simulink model "SpheroGigETracking"  (R2017b)
settings: Solver=FixedStepAuto  StartTime=0.0  StopTime=inf  RelTol=1e-3
undefined symbols (not defined in the file or in its folder): DeviceSpecific, gray, Rec, SDTV, videoinput
libraries: visionstatistics x2, dspnetwork x2, visionconversions x1, visiontextngfix x1, sphero_lib x1, imaqlib x1
settings Model: Creator=Michael  LastModifiedBy=Admin
settings CodeAppCC: StateflowObjectComments=on

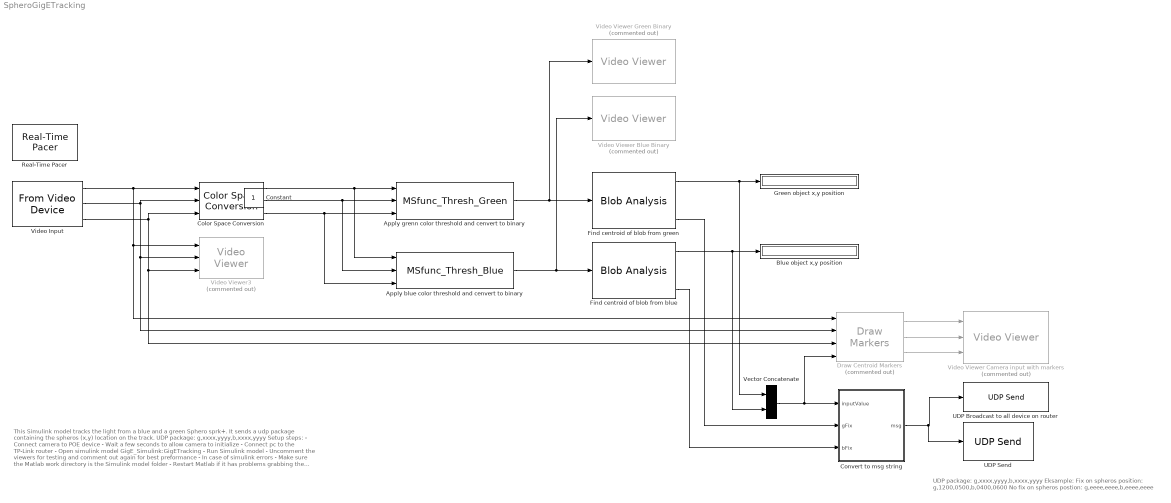
== system SpheroGigETracking ==
  note: This Simulink model tracks the light from a blue and
      | a green Sphero sprk+. It sends a udp package containing
      | the spheros (x,y) location on the track.
      | UDP package: g,xxxx,yyyy,b,xxxx,yyyy
      |
      | Setup steps:
      | - Connect camera to POE device
      | - Wait a few seconds to allow camera to initialize
      | - Connect pc to the TP-Link router
      | - Open simulink model GigE_Simulink:GigETracking
      | - Run Simulink model
      | - Uncomment the viewers for testing and comment out again
      | for best preformance
      |
      | - In case of simulink errors
      | - Make sure the Matlab work directory is the
      | Simulink model folder
      | - Restart Matlab if it has problems grabbing the video input
  note: UDP package: g,xxxx,yyyy,b,xxxx,yyyy
      |
      | Eksample:
      | Fix on spheros position: g,1200,0500,b,0400,0600
      | No fix on spheros postion: g,eeee,eeee,b,eeee,eeee
  Apply blue color threshold and cenvert to binary : M-S-Function  FunctionName=MSfunc_Thresh_Blue
  Apply grenn color threshold and cenvert to binary : M-S-Function  FunctionName=MSfunc_Thresh_Green
  Blue object x,y position : Display
  Color Space Conversion : visionconversions/Color Space  Conversion  conversion=Obsolete  conversionActive=R'G'B' to HSV  wp_str=D65  rec=Rec. 601 (SDTV)  sys=1125/60/2:1  imagePorts=Separate color signals
      settings: SourceProductName=Computer Vision System Toolbox
  Convert to msg string : MATLAB Function  TreatAsAtomicUnit=on
  Draw Centroid Markers : visiontextngfix/Draw Markers  Commented=on  shape=X-mark  size=25  fill=off  fillClrSource=Specify via dialog  display=White  intensity=200  color=[200 255 100]  opacity=0.6  viewport=Entire image  antialiasing=off  inType=Obsolete  imagePorts=Separate color signals  prodOutputMode=Binary point scaling  prodOutputWordLength=32  prodOutputFracLength=14  memoryMode=Specify word length  memoryWordLength=16  memoryFracLength=15  roundingMode=Floor  overflowMode=off
      settings: SourceProductName=Computer Vision System Toolbox  SourceProductBaseCode=VP
  Find centroid of blob from blue : visionstatistics/Blob Analysis  Tag=vipblks_row_conv  area=off  centroid=on  bBox=on  majorAxis=off  minorAxis=off  angle=off  eccentricity=off  equivDiameterSq=off  extent=off  perimeter=off  maxBlobs=1  warnIfNumBlobsExceeded=on  isCount=on  useMinArea=on  minArea=50  useMaxArea=on  maxArea=800  excludeBorderBlob=on  outDT=double  isOutVarDim=off  isFill=on  fillValues=0  conn=8  isLabel=off  outputMode=Binary point scaling  outputWordLength=32  outputFracLength=16  firstCoeffMode=Binary point scaling  firstCoeffWordLength=16  firstCoeffFracLength=14  secondCoeffMode=Binary point scaling  secondCoeffWordLength=32  secondCoeffFracLength=16  accumMode=Binary point scaling  accumWordLength=32  accumFracLength=0  prodOutputMode=Binary point scaling  prodOutputWordLength=32  prodOutputFracLength=16  roundingMode=Floor  overflowMode=off
      settings: SourceProductName=Computer Vision System Toolbox
  Find centroid of blob from green : visionstatistics/Blob Analysis  Tag=vipblks_row_conv  area=off  centroid=on  bBox=on  majorAxis=off  minorAxis=off  angle=off  eccentricity=off  equivDiameterSq=off  extent=off  perimeter=off  maxBlobs=1  warnIfNumBlobsExceeded=on  isCount=on  useMinArea=on  minArea=50  useMaxArea=on  maxArea=800  excludeBorderBlob=on  outDT=double  isOutVarDim=off  isFill=on  fillValues=0  conn=8  isLabel=off  outputMode=Binary point scaling  outputWordLength=32  outputFracLength=16  firstCoeffMode=Binary point scaling  firstCoeffWordLength=16  firstCoeffFracLength=14  secondCoeffMode=Binary point scaling  secondCoeffWordLength=32  secondCoeffFracLength=16  accumMode=Binary point scaling  accumWordLength=32  accumFracLength=0  prodOutputMode=Binary point scaling  prodOutputWordLength=32  prodOutputFracLength=16  roundingMode=Floor  overflowMode=off
      settings: SourceProductName=Computer Vision System Toolbox
  Green object x,y position : Display
  Real-Time Pacer : sphero_lib/Real-Time Pacer  simTimePerRealTime=1
  UDP Broadcast to all device on router : dspnetwork/UDP Send  remoteURL='192.168.1.11'  remotePort=55000  localURL='0.0.0.0'  localPortSource=Automatically determine  localPort=-1  sampletime=-1  blockPlatform=[]  separateLengthPort=0
      settings: SourceProductName=DSP System Toolbox  SourceProductBaseCode=DS
  UDP Send : dspnetwork/UDP Send  remoteURL='192.168.1.10'  remotePort=55000  localURL='0.0.0.0'  localPortSource=Automatically determine  localPort=-1  sampletime=-1  blockPlatform=HOST  separateLengthPort=0
      settings: SourceProductName=DSP System Toolbox  SourceProductBaseCode=DS
  Vector Concatenate : Concatenate  Mode=Multidimensional array
  Video Input : imaqlib/From Video Device  DeviceMenu=gige 1 (Mako G-192C (5087))  Device=gige 1 (Mako G-192C (5087))  ObjConstructor=videoinput('gige', 1)  VideoFormatMenu=BayerBG8  VideoFormat=BayerBG8  VideoSource=input1  ROIPosition=[400 700 400 400]  EnableHWTrigger=off  TriggerConfiguration=DeviceSpecific/DeviceSpecific  SampleTime=1/60  OutputPortsMode=Separate color signals  DataType=single  CanDoHWTrigger=yes  ReturnedColorSpace=rgb  BlockHandle=626.0002  ROIWidth=400  ROIHeight=400  ROIColumn=700  ROIRow=400  EngXMLPath=C:\Program Files\MATLAB\R2017b\toolbox\imaq\imaq\private  DevXMLPath=C:\ProgramData\MATLAB\SupportPackages\R2017b\toolbox\imaq\supportpackages\gige\adaptor\win64  EngLibPath=C:\Program Files\MATLAB\R2017b\toolbox\imaq\imaqblks\imaqmex\win64  ColorSpace=rgb  BayerSensorAlignment=grbg
      settings: SourceProductName=Image Acquisition Toolbox
  Video Viewer Blue Binary : VideoViewer  Commented=on  FigPos=[-128 1434 1280 882]
  Video Viewer Camera input with markers : VideoViewer  Commented=on  imagePorts=separate color signals  colormapValue=gray(256)  FigPos=[1 1022 1206 746]
  Video Viewer Green Binary : VideoViewer  Commented=on  FigPos=[-128 1434 1280 882]
  Video Viewer3 : VideoViewer  Commented=on  imagePorts=separate color signals  colormapValue=gray(256)  FigPos=[1 1022 1206 746]
  Constant : Constant  IOType=siggen
  wires:
  Color Space Conversion/1 -> Apply grenn color threshold and cenvert to binary/1, Apply blue color threshold and cenvert to binary/1
  Color Space Conversion/2 -> Apply grenn color threshold and cenvert to binary/2, Apply blue color threshold and cenvert to binary/2
  Color Space Conversion/3 -> Apply grenn color threshold and cenvert to binary/3, Apply blue color threshold and cenvert to binary/3
  Apply grenn color threshold and cenvert to binary/1 -> Find centroid of blob from green/1, Video Viewer Green Binary/1
  Find centroid of blob from green/1 -> Green object x,y position/1, Vector Concatenate/1
  Find centroid of blob from blue/1 -> Vector Concatenate/2, Blue object x,y position/1
  Vector Concatenate/1 -> Convert to msg string/1(inputValue), Draw Centroid Markers/4
  Video Input/2 -> Draw Centroid Markers/2, Video Viewer3/2, Color Space Conversion/2
  Video Input/3 -> Draw Centroid Markers/3, Video Viewer3/3, Color Space Conversion/3
  Draw Centroid Markers/1 -> Video Viewer Camera input with markers/1
  Draw Centroid Markers/2 -> Video Viewer Camera input with markers/2
  Draw Centroid Markers/3 -> Video Viewer Camera input with markers/3
  Video Input/1 -> Draw Centroid Markers/1, Video Viewer3/1, Color Space Conversion/1
  Convert to msg string/1(msg) -> UDP Send/1, UDP Broadcast to all device on router/1
  Apply blue color threshold and cenvert to binary/1 -> Find centroid of blob from blue/1, Video Viewer Blue Binary/1
  Find centroid of blob from green/3 -> Convert to msg string/2(gFix)
  Find centroid of blob from blue/3 -> Convert to msg string/3(bFix)

== matlab function SpheroGigETracking/Convert to msg string ==
  data: inputValue input; msg output; gFix input; bFix input
function msg = fcn(inputValue,gFix,bFix)
    %r = [inputValue(1) inputValue(4)];
    g = [inputValue(1) inputValue(3)];
    b = [inputValue(2) inputValue(4)];
    greenFix = gFix;
    blueFix = bFix;
    
    msgToSend = zeros(1,23);
    idx = 1;
    
%     coorR = uint16(r);
%     msgR = IndividualString('r', coorR);
%     for i=1:11
%         msgToSend(idx) = msgR(i);
%         idx = idx + 1;
%     end
%     msgToSend(idx) = ',';
%     idx = idx + 1;
    
    coorG = uint16(g);
    msgG = IndividualString('g', coorG, greenFix);
    for i=1:11
        msgToSend(idx) = msgG(i);
        idx = idx + 1;
    end
    msgToSend(idx) = ',';
    idx = idx + 1;
    
    coorB = uint16(b);
    msgB = IndividualString('b', coorB, blueFix);
    for i=1:11
        msgToSend(idx) = msgB(i);
        idx = idx + 1;
    end
    
    msg = uint8(msgToSend);
    
end

function msgIndividual = IndividualString(color, Coord, fix)
    spheroFix = fix;
    xIdx = Coord(1);
    yIdx = Coord(2);
    msgIndividual = zeros(1,11);
    msgIdx = 1;    
    msgIndividual(msgIdx) = color;
    msgIdx = msgIdx + 1;
    msgIndividual(msgIdx) = ':';
    msgIdx = msgIdx + 1;
    
    xIdxStr = int2str(xIdx);
    lenX = length(xIdxStr);
    if(spheroFix)
        for i = 0:3
            if(lenX < (4-i))
                msgIndividual(msgIdx) = '0';
            else
                msgIndividual(msgIdx) = xIdxStr(lenX - (3-i));
            end
            msgIdx = msgIdx + 1;
        end
        msgIndividual(msgIdx) = ':';
        msgIdx = msgIdx + 1;
        yIdxStr = int2str(yIdx);
        lenY = length(yIdxStr);
        for i = 0:3
            if(lenY < (4-i))
                msgIndividual(msgIdx) = '0';
            else
                msgIndividual(msgIdx) = yIdxStr(lenY - (3-i));
            end
            msgIdx = msgIdx + 1;
        end
    else
        for i = 0:3
            msgIndividual(msgIdx) = 'e';
            msgIdx = msgIdx + 1;
        end
        msgIndividual(msgIdx) = ':';
        msgIdx = msgIdx + 1;
        for i = 0:3
            msgIndividual(msgIdx) = 'e';
            msgIdx = msgIdx + 1;
        end
    end
end
